simulink model "otfs"  (R2025a)
settings: Solver=VariableStepAuto  StartTime=0.0  StopTime=1  RelTol=1e-3
values from neighbouring files (symbols this model uses):
  chanParams =     [OFDM_DATA.mat]
  fsamp = M * df    (= 30720000)    [DDBDM.m]    (also in tdl_chanel.m = 960000)
  G = G + diag(vec, -l)    [DDBDM.m]    (also in tdl_chanel.m)
  M = 256    [DDBDM.m]    (also in OFDM_DATA.mat; ofdm_code.m = modSpec.M; tdl_chanel.m = 64)
  Meff = M + padLen    (= 396)    [DDBDM.m]    (also in tdl_chanel.m = 74)
  N = 16    [DDBDM.m]    (also in tdl_chanel.m = 30)
  n0 = EsQPSK / (10^(SNRdB/10))    [DDBDM.m]    (also in tdl_chanel.m = Es/(10^(SNRdB/10)))
  padLen = 140    [DDBDM.m]    (also in tdl_chanel.m = 10)
  SNRdB = SNRvec(idxS)    [DDBDM.m]    (also in OFDM_DATA.mat = 30; ofdm_code.m = SNRvec(iS); tdl_chanel.m = 40)
  T = ((M + padLen) / (M * df))    (= 1.2890625e-05)    [DDBDM.m]    (also in tdl_chanel.m = 7.70833333333e-05)
libraries: dspxfrm3 x2, commdigbbndpm3 x2, commsink2 x1, commrandsrc3 x1, dspstat3 x1
settings Model: Creator=santi  LastModifiedBy=santi

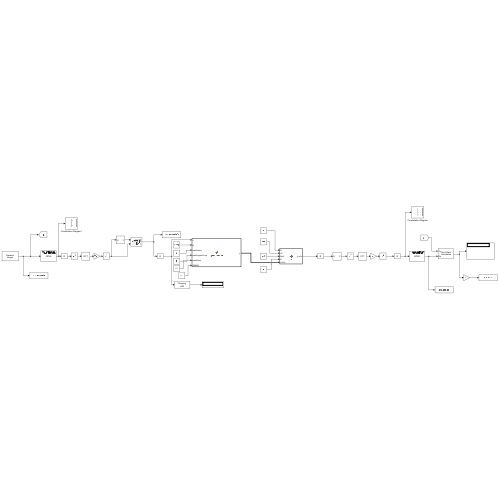
[thumbnail: Simulink's stored preview of the top-level diagram]
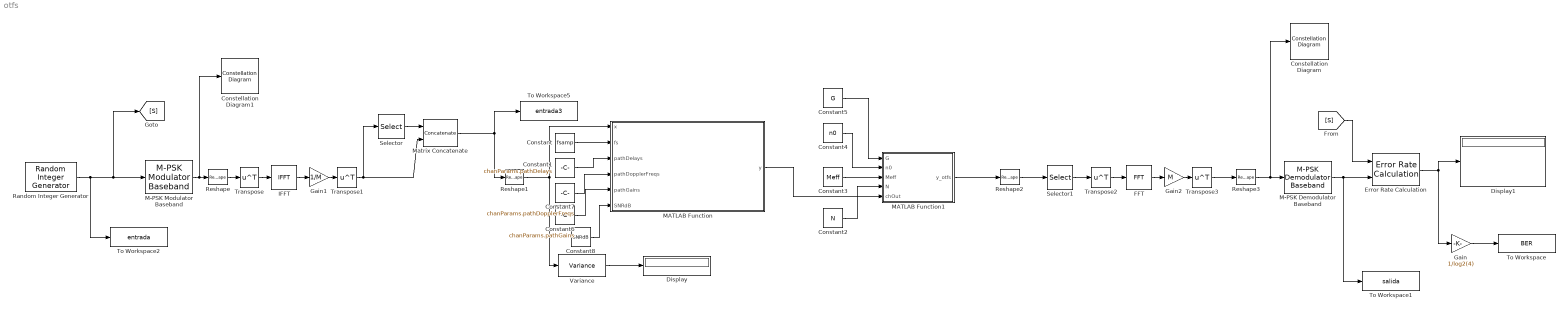
== system otfs ==
  Constant : Constant  Value=fsamp
  Constant1 : Constant  Value=chanParams.pathDelays  VectorParams1D=off
  Constant2 : Constant  Value=N
  Constant3 : Constant  Value=Meff
  Constant4 : Constant  Value=n0
  Constant5 : Constant  Value=G  VectorParams1D=off
  Constant6 : Constant  Value=chanParams.pathGains  VectorParams1D=off
  Constant7 : Constant  Value=chanParams.pathDopplerFreqs  VectorParams1D=off
  Constant8 : Constant  Value=SNRdB  VectorParams1D=off
  Constellation Diagram : ConstellationDiagram  WindowPosition=[340.000000,60.000000,600.000000,600.000000,]  Visible=on  ScopeFrameLocation=window  SymbolsToDisplaySource=Property  SymbolsToDisplay=10000  DefaultConfigurationName=comm.scopes.ConstellationDiagramBlockCfg
  Constellation Diagram1 : ConstellationDiagram  WindowPosition=[340.000000,60.000000,600.000000,600.000000,]  Visible=on  ScopeFrameLocation=window  SymbolsToDisplaySource=Property  SymbolsToDisplay=10000  DefaultConfigurationName=comm.scopes.ConstellationDiagramBlockCfg
  Display : Display
  Display1 : Display
  Error Rate Calculation : commsink2/Error Rate Calculation  N=0  st_delay=0  cp_mode=Entire frame  subframe=[]  PMode=Port  WsName=ErrorVec  RsMode2=off  stop=off  numErr=100  maxBits=1e6
      settings: LibrarySourceBlock=|
      | commhdlsink/Error Rate
      | Calculation
  FFT : dspxfrm3/FFT  FFTImplementation=Auto  CompMethod=Table lookup  TableOpt=NEW  TableOptActive=Speed  BitRevOrder=off  Normalize=off  InheritFFTLength=on  FFTLength=64  WrapInput=on  roundingMode=Ceiling  overflowMode=off  firstCoeffDataTypeStr=Inherit: Same word length as input  firstCoeffLastDataTypeStr=Inherit: Same word length as input  outputMin=[]  outputMax=[]
  Gain : Gain  Gain=1/log2(4)
  Gain1 : Gain  Gain=1/M
  Gain2 : Gain  Gain=M
  IFFT : dspxfrm3/IFFT  FFTImplementation=Auto  CompMethod=Table lookup  TableOpt=NEW  TableOptActive=Speed  BitRevOrder=off  cs_in=off  Normalize=on  InheritFFTLength=on  FFTLength=64  WrapInput=on  mode=Real  outSamplingMode=Sample based  roundingMode=Ceiling  overflowMode=off  firstCoeffDataTypeStr=Inherit: Same word length as input  firstCoeffLastDataTypeStr=Inherit: Same word length as input  outputMin=[]  outputMax=[]
  M-PSK Demodulator Baseband : commdigbbndpm3/M-PSK Demodulator Baseband  M=4  OutType=Integer  DecType=Hard decision  VarSource=Dialog  Variance=1  Dec=Gray  Mapping=[0:7]  Ph=pi/4  outDtype1=Inherit via internal rule  outDtype2=Inherit via internal rule  derotateFactorWordLen=16  derotateFactorDataTypeStr=Inherit: Same word length as input  derotateFactorLastDataTypeStr=Inherit: Same word length as input
      settings: LibrarySourceBlock=|
      | commhdldigbbndpm/M-PSK
      | Demodulator
      | Baseband
  M-PSK Modulator Baseband : commdigbbndpm3/M-PSK Modulator Baseband  M=4  InType=Integer  Enc=Gray  Mapping=[0:7]  Ph=pi/4  outDtype=double  outWordLen=16  outUDDataType=sfix(16)  outFracLenMode=Best precision  outFracLen=15  outDataTypeStr=double  outLastDataTypeStr=double
      settings: LibrarySourceBlock=|
      | commhdldigbbndpm/M-PSK
      | Modulator
      | Baseband
  MATLAB Function : MATLAB Function  TreatAsAtomicUnit=on
  MATLAB Function1 : MATLAB Function  TreatAsAtomicUnit=on
  Matrix Concatenate : Concatenate  Mode=Multidimensional array
  Random Integer Generator : commrandsrc3/Random Integer Generator  SetSize=4  SeedSource=Parameter  Seed=37  SampleTime=T  SamplesPerFrame=M*N  OutputDataType=double  SimulateUsing=Interpreted execution
  Reshape : Reshape  OutputDimensionality=Customize  OutputDimensions=[M,N]
  Reshape1 : Reshape  OutputDimensionality=Customize  OutputDimensions=[Meff*N,1]
  Reshape2 : Reshape  OutputDimensionality=Customize  OutputDimensions=[Meff,N]
  Reshape3 : Reshape  OutputDimensionality=Customize  OutputDimensions=[M*N,1]
  Selector : Selector  NumberOfDimensions=2  InputPortWidth=3  IndexOptions=Index vector (dialog),Select all  Indices=[M-padLen+1:M],1  OutputSizes=1,1
  Selector1 : Selector  NumberOfDimensions=2  InputPortWidth=3  IndexOptions=Index vector (dialog),Select all  Indices=[padLen+1:Meff],1  OutputSizes=1,1
  To Workspace : ToWorkspace  VariableName=BER  SaveFormat=Timeseries  SampleTime=-1
  To Workspace1 : ToWorkspace  VariableName=salida  SaveFormat=Timeseries  SampleTime=-1
  To Workspace2 : ToWorkspace  VariableName=entrada  SaveFormat=Timeseries  SampleTime=-1
  To Workspace5 : ToWorkspace  VariableName=entrada3  SaveFormat=Timeseries  SampleTime=-1
  Transpose{,1..3} (4 alike) : Math  Operator=transpose
  Variance : dspstat3/Variance  run=on  InputProcessing=Columns as channels (frame based)  reset_popup=None  directionMode=Each column  dimension=1  roiEnable=off  roiType=Rectangles  roiPortion=Entire ROI  roiOutput=Individual statistics for each ROI  roiFlag=off  roundingMode=Floor  overflowMode=off
  wires:
  Variance/1 -> Display/1
  Random Integer Generator/1 -> To Workspace2/1, [S], M-PSK Modulator Baseband/1
  M-PSK Modulator Baseband/1 -> Constellation Diagram1/1, Reshape/1
  M-PSK Demodulator Baseband/1 -> To Workspace1/1, Error Rate Calculation/2
  Error Rate Calculation/1 -> Display1/1, Gain/1
  Gain/1 -> To Workspace/1
  [S] -> Error Rate Calculation/1
  Reshape/1 -> Transpose/1
  Transpose/1 -> IFFT/1
  Transpose1/1 -> Matrix Concatenate/2, Selector/1
  Selector/1 -> Matrix Concatenate/1
  Matrix Concatenate/1 -> Reshape1/1, To Workspace5/1
  Reshape1/1 -> Variance/1, MATLAB Function/1(x)
  Reshape2/1 -> Selector1/1
  Selector1/1 -> Transpose2/1
  Transpose2/1 -> FFT/1
  IFFT/1 -> Gain1/1
  Gain1/1 -> Transpose1/1
  FFT/1 -> Gain2/1
  Gain2/1 -> Transpose3/1
  Transpose3/1 -> Reshape3/1
  Constant/1 -> MATLAB Function/2(fs)
  Constant2/1 -> MATLAB Function1/4(N)
  Constant3/1 -> MATLAB Function1/3(Meff)
  Constant4/1 -> MATLAB Function1/2(n0)
  Constant5/1 -> MATLAB Function1/1(G)
  MATLAB Function1/1(y_otfs) -> Reshape2/1
  Constant1/1 -> MATLAB Function/3(pathDelays)
  Constant6/1 -> MATLAB Function/5(pathGains)
  Constant7/1 -> MATLAB Function/4(pathDopplerFreqs)
  MATLAB Function/1(y) -> MATLAB Function1/5(chOut)
  Reshape3/1 -> Constellation Diagram/1, M-PSK Demodulator Baseband/1
  Constant8/1 -> MATLAB Function/6(SNRdB)

== matlab function otfs/MATLAB Function1 ==
  data: G input; y_otfs output; n0 input; Meff input; N input; chOut input
function y_otfs = equalization(G,n0,Meff,N,chOut)
    rxWindow = chOut(1:Meff*N);
    y_otfs = ((G'*G)+n0*eye(Meff*N)) \ (G'*rxWindow);

== matlab function otfs/MATLAB Function ==
  data: x input; y output [0..10000]; fs input; pathDelays input; pathDopplerFreqs input; pathGains input; SNRdB input
function y = dopplerChannel(x,fs,pathDelays,pathDopplerFreqs,pathGains,SNRdB)
    % Form an output vector y comprising paths of x with different
    % delays, Dopplers, and complex gains
    numPaths = length(pathDelays);
    maxPathDelay = max(pathDelays);
    txOutSize = length(x);
    
    y = complex(zeros(txOutSize+maxPathDelay,1));
    
    for k = 1:numPaths
        pathOut = complex(zeros(txOutSize+maxPathDelay,1));

        % Doppler
        pathShift = frequencyOffset(x,fs,pathDopplerFreqs(k));
    
        % Delay and gain
        pathOut(1+pathDelays(k):pathDelays(k)+txOutSize) = ...
            pathShift * pathGains(k);
            
        y = y + pathOut;
    end
    y=awgn(y,SNRdB,'measured');
end
